simulink model "Problem4_Filter_ReferenceModel"  (R2020b)
settings: Solver=VariableStepAuto  StartTime=0.0  StopTime=10  MaxStep=0.01  RelTol=1e-3
settings Model: Creator=vigne  LastModifiedBy=vigne
settings DataIOCC: SaveOutput=off  SaveTime=off

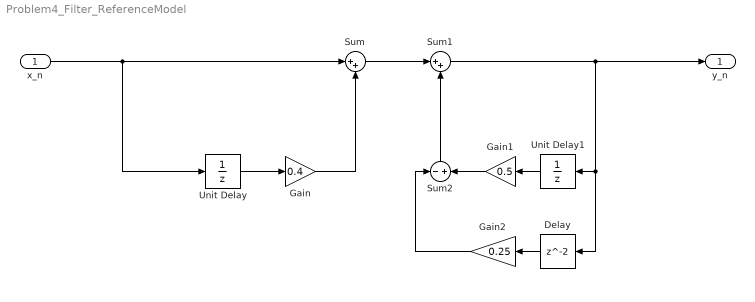
== system Problem4_Filter_ReferenceModel ==
  x_n : Inport  OutDataTypeStr=double  PortDimensions=1  SampleTime=0
  Delay : Delay
  Gain : Gain  Gain=0.4
  Gain1 : Gain  Gain=0.5
  Gain2 : Gain  Gain=0.25
  Sum : Sum  Inputs=|++
  Sum1 : Sum  Inputs=|++
  Sum2 : Sum  Inputs=-+
  Unit Delay : UnitDelay  SampleTime=-1  HasFrameUpgradeWarning=on
  Unit Delay1 : UnitDelay  SampleTime=-1  HasFrameUpgradeWarning=on
  y_n : Outport  OutDataTypeStr=double  PortDimensions=1  SampleTime=0
  wires:
  Sum2/1 -> Sum1/2
  Sum1/1 -> Delay/1, Unit Delay1/1, y_n/1
  x_n/1 -> Unit Delay/1, Sum/1
  Delay/1 -> Gain2/1
  Gain2/1 -> Sum2/1
  Gain1/1 -> Sum2/2
  Unit Delay/1 -> Gain/1
  Unit Delay1/1 -> Gain1/1
  Sum/1 -> Sum1/1
  Gain/1 -> Sum/2
